simulink model "nelinearni"  (R2019b)
settings: Solver=VariableStepAuto  StartTime=0.0  StopTime=10.0  RelTol=1e-3
settings Model: Creator=Já  LastModifiedBy=Já

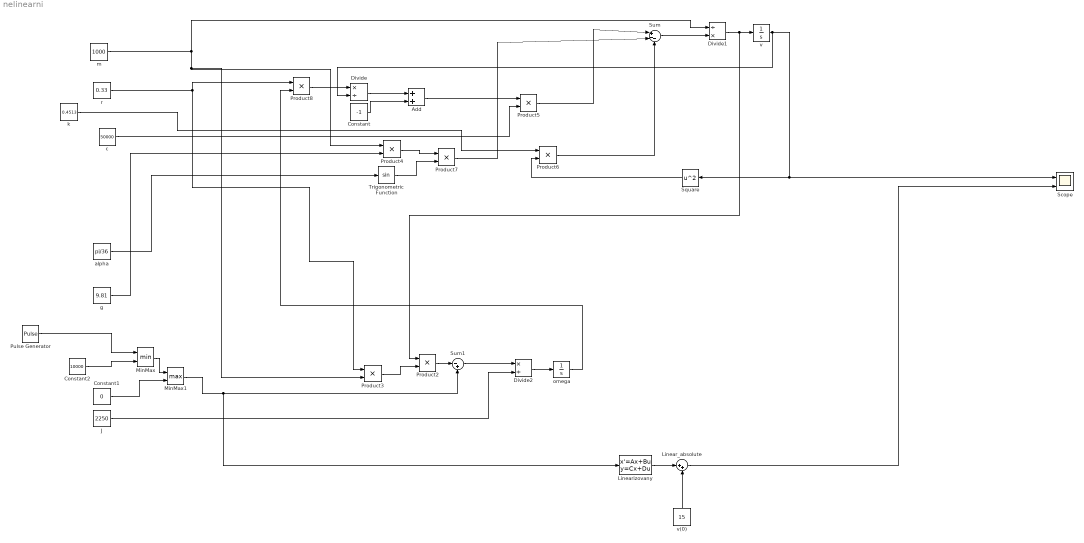
== system nelinearni ==
  Add : Sum
  Constant : Constant  Value=-1
  Constant1 : Constant  Value=0
  Constant2 : Constant  Value=10000
  Divide : Product  Inputs=*/
  Divide1 : Product  Inputs=/*
  Divide2 : Product  Inputs=*/
  J : Constant  Value=2250
  Linear_absolute : Sum  Inputs=|++
  Linearizovany : StateSpace  A=[-3.4106 1.1; 0.5043 0.16133]  B=[0; 1/2250]  C=[1 0]  D=0  InitialCondition=[0 ; 0]
  MinMax : MinMax  Inputs=2
  MinMax1 : MinMax  Function=max  Inputs=2
  Product{2..8} (7 alike) : Product
  Pulse Generator : DiscretePulseGenerator  PulseType=Time based  Amplitude=500  Period=1  PulseWidth=0.01
  Scope : Scope  NumInputPorts=2
  Square : Math  Operator=square  SignedPower=off  SaturateOnIntegerOverflow=on
  Sum : Sum  Inputs=|+--
  Sum1 : Sum  Inputs=|-+
  Trigonometric Function : Trigonometry
  alpha : Constant  Value=pi/36
  c : Constant  Value=50000
  g : Constant  Value=9.81
  "k " : Constant  Value=0.4513
  m : Constant  Value=1000
  omega : Integrator  InitialCondition=46.3241
  r : Constant  Value=0.33
  v : Integrator  InitialCondition=15
  v(0) : Constant  Value=15
  wires:
  v/1 -> Divide/2, Square/1, Scope/1
  Divide1/1 -> Product2/1, v/1
  Divide2/1 -> omega/1
  Sum/1 -> Divide1/2
  J/1 -> Divide2/2
  Sum1/1 -> Divide2/1
  Product2/1 -> Sum1/1
  Product3/1 -> Product2/2
  r/1 -> Product8/1, Product3/1
  m/1 -> Divide1/1, Product3/2, Product4/1
  omega/1 -> Product8/2
  Product8/1 -> Divide/1
  Divide/1 -> Add/1
  Constant/1 -> Add/2
  g/1 -> Product4/2
  Trigonometric Function/1 -> Product7/2
  Product4/1 -> Product7/1
  Product7/1 -> Sum/2
  "k "/1 -> Product6/1
  Add/1 -> Product5/1
  c/1 -> Product5/2
  Product5/1 -> Sum/1
  Product6/1 -> Sum/3
  Square/1 -> Product6/2
  alpha/1 -> Trigonometric Function/1
  MinMax/1 -> MinMax1/1
  MinMax1/1 -> Linearizovany/1, Sum1/2
  Constant2/1 -> MinMax/2
  Pulse Generator/1 -> MinMax/1
  Constant1/1 -> MinMax1/2
  v(0)/1 -> Linear_absolute/2
  Linearizovany/1 -> Linear_absolute/1
  Linear_absolute/1 -> Scope/2
